simulink library "Weather_Simple_Model"  (R2018b)
settings: Solver=ode45  StartTime=0.0  StopTime=10.0  RelTol=1e-3  EnableMultiTasking=on
libraries: carnot x4, simulink x1
settings Model: Creator=lena.frank  LastModifiedBy=drhf
settings DataIOCC: LimitDataPoints=on  SaveFormat=Array  SignalLoggingSaveFormat=ModelDataLogs
settings OptimizationCC: ExpressionDepthLimit=2147483647  LifeSpan=inf
settings DebuggingCC: UnderspecifiedInitializationDetection=Classic  MergeDetectMultiDrivingBlocksExec=none  SolverPrmCheckMsg=warning  FcnCallInpInsideContextMsg=warning  StateNameClashWarn=warning  SFUnexpectedBacktrackingDiag=warning  SFNoUnconditionalDefaultTransitionDiag=warning  SFExecutionAtInitializationDiag=none
settings HardwareCC: ProdBitPerPointer=32  ProdBitPerSizeT=32  ProdBitPerPtrDiffT=32  ProdLargestAtomicFloat=None  ProdIntDivRoundTo=Undefined  ProdEndianess=Unspecified  ProdWordSize=32  ProdHWDeviceType=32-bit Generic
settings ModelReferenceCC: PropagateSignalLabelsOutOfModel=off
settings SFSimCC: SimUseLocalCustomCode=off
settings RTWCC: RTWUseLocalCustomCode=off
settings CodeAppCC: StateflowObjectComments=on
settings GRTTargetCC: TargetLangStandard=C89/C90 (ANSI)  GeneratePreprocessorConditionals=Disable all  CombineOutputUpdateFcns=off  GRTInterface=on
settings ConfigComp: CovMetricSettings=dw  CovHtmlReporting=on  CovSaveCumulativeToWorkspaceVar=on  CovSaveSingleToWorkspaceVar=on  CovExternalEMLEnable=off

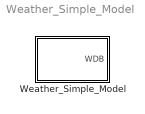
== system Weather_Simple_Model ==
  Weather_Simple_Model : Subsystem  mask(Weather Simple Model){Ibn=900, Idg=100, tamb=5, deltaTsky=-6, rh=50, precip=10e-3/24/3600           % 10 mm in 24 h, cloud=0.125, p=1013e2, vw=1, wdir=270, lat=50, longi=0, timezone=0, colangle=0, colazi=0, colrot=0}
      mask prompts: Ibn "Maximum beam radiation on normal surface in W/m²"; Idg "Maximum diffuse radiation on horizontal surface in W/m²"; tamb "Ambient temperature in °C"; deltaTsky "Offset for sky temperature in K (usually -6K)"; rh "Relative humidity in %"; precip "Rainfall (precipitation) in m/s"; cloud "Cloud index in (0..1)"; p "Air pressure in Pa"; vw "Wind speed in m/s"; wdir "Wind direction in ° (0° = North, 90° = East)"; lat "Latitude in degree (-90..+90, North postive)"; longi "Longitude in degree (-180..+180, West postive)"; timezone "Longitude of timezone in degree (-180..+180, West postive)"; colangle "Slope of surface (0° = horizontal) [degree]"; colazi "Azimuth of surface (0° = south, -90° = east) [degree]"; colrot "Rotation angle of surface [degree]"
      mask help:
      | Create a simple, mostly constant weather data bus (WDB).
      | The solar radiation corresponds to clear sky conditions.
      mask Help: web(fullfile(path_carnot('help'),'Weather_Simple_Model.html'),'-helpbrowser')
      mask TypeOptions lat: Solar_Position/lati
      mask TypeOptions longi: Solar_Position/longi
      mask TypeOptions timezone: Solar_Position/timezone
      mask TypeOptions colangle: Fixed_Surface/colangle
      mask TypeOptions colazi: Fixed_Surface/colazi
      mask TypeOptions colrot: Fixed_Surface/colrot
      mask DialogControl ParameterTabVar01 Prompt: Weather
      mask DialogControl ParameterTabVar0 Prompt: Geography
      mask DialogControl Container6 Prompt: Surface orientation
      mask Display:
      | plot(0,0,100,100, ...
      |     [10,7,10,20,30,23,25,40,54,56,50,60,70,73,70,60,20,10]*0.8+5, ...
      |     [15,24,34,40,35,42,50,55,50,42,35,40,34,24,15,10,10,15], ...
      |     [70,60,60,70,80,90,90,80,70]*0.7-30,...
      |     [90,80,70,60,60,70,80,90,90],...
      |     [75,75]*0.7-30,[91,97],...
      |     [75,75]*0.7-30,[52,58],...
      |     [58,52]*0.7-30,[75,75],...
      |     [98,91]*0.7-30,[75,75],...
      |     [63,58]*0.7-30,[63,57],...
      |     [92,86]*0.7-30,[92,87],...
      |     [63,58]*0.7-30,[85,92],...
      |     [92,86]*0.7-30,[57,64])

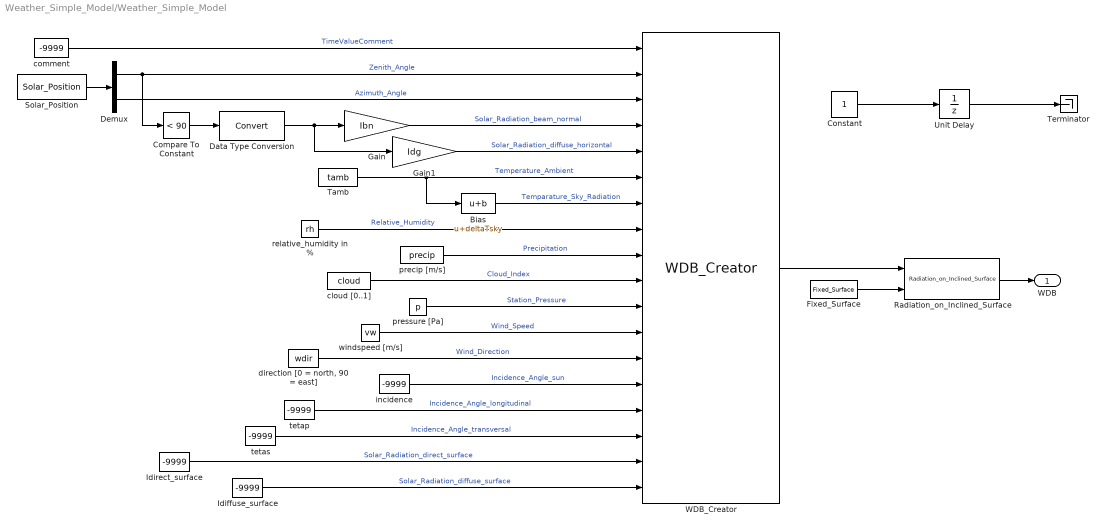
== system Weather_Simple_Model/Weather_Simple_Model ==
  Bias : Bias  Bias=deltaTsky
  Compare To Constant : simulink/Logic and Bit Operations/Compare To Constant  relop=<  const=90  OutDataTypeStr=uint8
  Constant : Constant
  Data Type Conversion : DataTypeConversion
  Demux : Demux  Outputs=2
  Fixed_Surface : carnot/Weather/Fixed_Surface  colangle=colangle  colazi=colazi  colrot=colrot
      settings: SourceProductName=Carnot
  Gain : Gain  Gain=Ibn
  Gain1 : Gain  Gain=Idg
  Idiffuse_surface : Constant  Value=-9999
  Idirect_surface : Constant  Value=-9999
  Radiation_on_Inclined_Surface : carnot/Weather/Radiation_on_Inclined_Surface  sky=Perez 1990  reflect=0.2
      settings: SourceProductName=Carnot
  Solar_Position : carnot/Basic/Weather_and_Sun/Solar_Position  lati=lat  longi=longi  timezone=timezone
      settings: SourceProductName=Carnot
  Tamb : Constant  Value=tamb
  Terminator : Terminator
  Unit Delay : UnitDelay  SampleTime=3600
  WDB_Creator : carnot/Basic/Weather_and_Sun/WDB_Creator
      settings: SourceProductName=Carnot
  cloud [0..1] : Constant  Value=cloud
  comment : Constant  Value=-9999
  "direction [0 = north, 90 = east]" : Constant  Value=wdir
  incidence : Constant  Value=-9999
  precip [m/s] : Constant  Value=precip
  pressure [Pa] : Constant  Value=p
  relative_humidity in % : Constant  Value=rh
  tetap : Constant  Value=-9999
  tetas : Constant  Value=-9999
  windspeed [m/s] : Constant  Value=vw
  WDB : Outport
  wires:
  Unit Delay/1 -> Terminator/1
  Constant/1 -> Unit Delay/1
  Data Type Conversion/1 -> Gain/1, Gain1/1
  Idiffuse_surface/1 -> WDB_Creator/18  "Solar_Radiation_diffuse_surface"
  Idirect_surface/1 -> WDB_Creator/17  "Solar_Radiation_direct_surface"
  tetas/1 -> WDB_Creator/16  "Incidence_Angle_transversal"
  tetap/1 -> WDB_Creator/15  "Incidence_Angle_longitudinal"
  incidence/1 -> WDB_Creator/14  "Incidence_Angle_sun"
  "direction [0 = north, 90 = east]"/1 -> WDB_Creator/13  "Wind_Direction"
  windspeed [m/s]/1 -> WDB_Creator/12  "Wind_Speed"
  pressure [Pa]/1 -> WDB_Creator/11  "Station_Pressure"
  cloud [0..1]/1 -> WDB_Creator/10  "Cloud_Index"
  precip [m/s]/1 -> WDB_Creator/9  "Precipitation"
  relative_humidity in %/1 -> WDB_Creator/8  "Relative_Humidity"
  Bias/1 -> WDB_Creator/7  "Temparature_Sky_Radiation"
  Tamb/1 -> Bias/1, WDB_Creator/6  "Temperature_Ambient"
  Gain1/1 -> WDB_Creator/5  "Solar_Radiation_diffuse_horizontal"
  Compare To Constant/1 -> Data Type Conversion/1
  Demux/2 -> WDB_Creator/3  "Azimuth_Angle"
  Demux/1 -> Compare To Constant/1, WDB_Creator/2  "Zenith_Angle"
  comment/1 -> WDB_Creator/1  "TimeValueComment"
  Solar_Position/1 -> Demux/1
  Gain/1 -> WDB_Creator/4  "Solar_Radiation_beam_normal"
  Fixed_Surface/1 -> Radiation_on_Inclined_Surface/2
  Radiation_on_Inclined_Surface/1 -> WDB/1
  WDB_Creator/1 -> Radiation_on_Inclined_Surface/1
